simulink model "helicopter_again"  (R2021a)
settings: Solver=VariableStepAuto  StartTime=0.0  StopTime=10  RelTol=1e-3
values from neighbouring files (symbols this model uses):
  A = [-0.4 0 -0.01; 1 0 0; -1.4 9.8 -0.02]    [heli_again.m]
  B = [6.3; 0; 9.8]    [heli_again.m]
  C = [0 0 1]    [heli_again.m]
  sample_time = 0.1    [heli_again.m]
undefined symbols (not defined in the file or in its folder): K_integrate, K_integrate_discretized
settings Model: Creator=davidrico  LastModifiedBy=davidrico

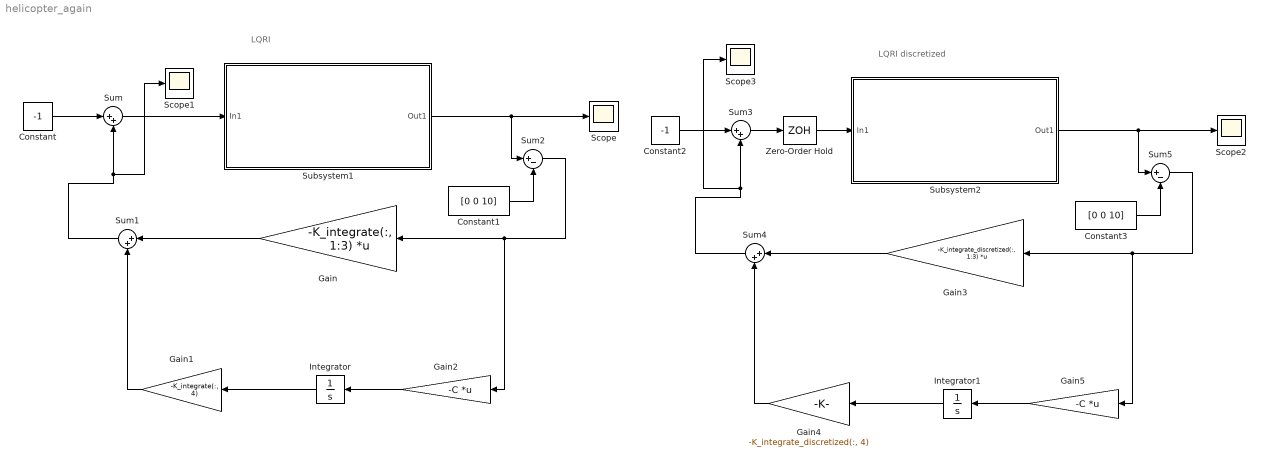
== system helicopter_again ==
  note: LQRI
  note: LQRI discretized
  Constant : Constant  Value=-1
  Constant1 : Constant  Value=[0 0 10]
  Constant2 : Constant  Value=-1
  Constant3 : Constant  Value=[0 0 10]
  Gain : Gain  Gain=-K_integrate(:, 1:3)  Multiplication=Matrix(K*u) (u vector)
  Gain1 : Gain  Gain=-K_integrate(:, 4)
  Gain2 : Gain  Gain=-C  Multiplication=Matrix(K*u) (u vector)
  Gain3 : Gain  Gain=-K_integrate_discretized(:, 1:3)  Multiplication=Matrix(K*u) (u vector)
  Gain4 : Gain  Gain=-K_integrate_discretized(:, 4)
  Gain5 : Gain  Gain=-C  Multiplication=Matrix(K*u) (u vector)
  Integrator : Integrator  InitialCondition=10
  Integrator1 : Integrator
  Scope{,1..3} (4 alike) : Scope
  Subsystem1 : Subsystem
  Subsystem2 : Subsystem
  Sum{,1,3..4} (4 alike) : Sum  Inputs=|++
  Sum2 : Sum  Inputs=|+-
  Sum5 : Sum  Inputs=|+-
  Zero-Order Hold : ZeroOrderHold  SampleTime=sample_time
  wires:
  Subsystem1/1(Out1) -> Sum2/1, Scope/1
  Sum/1 -> Subsystem1/1(In1)
  Constant/1 -> Sum/1
  Integrator/1 -> Gain1/1
  Gain/1 -> Sum1/1
  Sum1/1 -> Scope1/1, Sum/2
  Gain1/1 -> Sum1/2
  Gain2/1 -> Integrator/1
  Sum2/1 -> Gain2/1, Gain/1
  Constant1/1 -> Sum2/2
  Sum3/1 -> Zero-Order Hold/1
  Constant3/1 -> Sum5/2
  Sum5/1 -> Gain5/1, Gain3/1
  Gain4/1 -> Sum4/2
  Gain5/1 -> Integrator1/1
  Gain3/1 -> Sum4/1
  Subsystem2/1(Out1) -> Sum5/1, Scope2/1
  Sum4/1 -> Scope3/1, Sum3/2
  Constant2/1 -> Sum3/1
  Integrator1/1 -> Gain4/1
  Zero-Order Hold/1 -> Subsystem2/1(In1)

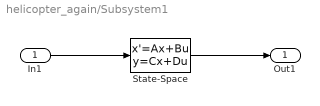
== system helicopter_again/Subsystem1 ==
  In1 : Inport
  State-Space : StateSpace  A=A  B=B  C=eye(3)  D=zeros(3,1)  InitialCondition=[1; 1; 1]
  Out1 : Outport
  wires:
  In1/1 -> State-Space/1
  State-Space/1 -> Out1/1

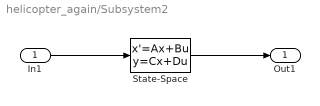
== system helicopter_again/Subsystem2 ==
  In1 : Inport
  State-Space : StateSpace  A=A  B=B  C=eye(3)  D=zeros(3,1)  InitialCondition=[1; 1; 1]
  Out1 : Outport
  wires:
  In1/1 -> State-Space/1
  State-Space/1 -> Out1/1
